simulink model "PWM_controller"  (R2014b)
settings: Solver=FixedStepDiscrete  StartTime=0.0  StopTime=150000  FixedStep=1  RelTol=1e-3
libraries: simulink x1
settings Model: FPTRunName=FPA_Reference  SimulationMode=rapid-accelerator  Creator=variable  LastModifiedBy=maclab3
settings DataIOCC: SaveOutput=off  SignalLogging=off  DSMLogging=off  SaveTime=off
settings OptimizationCC: BlockReduction=off  ConditionallyExecuteInputs=off  InlineParams=on
settings DebuggingCC: SignalRangeChecking=warning  AlgebraicLoopMsg=error  ParameterDowncastMsg=warning  ParameterOverflowMsg=warning  LoggingUnavailableSignals=none
settings HardwareCC: ProdHWDeviceType=ASIC/FPGA->ASIC/FPGA  TargetLongLongMode=on  TargetIntDivRoundTo=Zero  TargetEndianess=LittleEndian  TargetHWDeviceType=MATLAB Host  ProdEqTarget=off

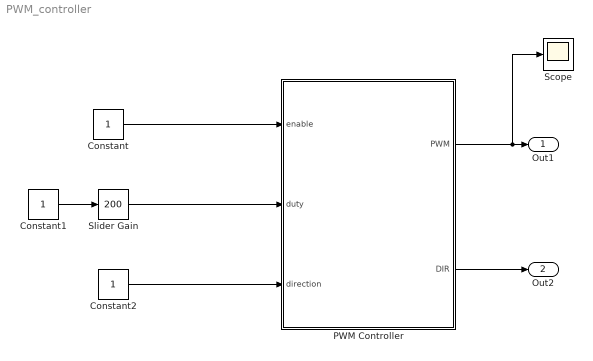
== system PWM_controller ==
  Constant : Constant  OutDataTypeStr=boolean  SampleTime=-1
  Constant1 : Constant  OutDataTypeStr=uint8  SampleTime=-1
  Constant2 : Constant  OutDataTypeStr=boolean  SampleTime=-1
  PWM Controller : Subsystem  TreatAsAtomicUnit=on
  Scope : Scope
  Slider Gain : simulink/Math Operations/Slider Gain  low=0  gain=200  high=255
  Out1 : Outport
  Out2 : Outport  Port=2
  wires:
  Constant/1 -> PWM Controller/1(enable)
  Constant1/1 -> Slider Gain/1
  Constant2/1 -> PWM Controller/3(direction)
  Slider Gain/1 -> PWM Controller/2(duty)
  PWM Controller/1(PWM) -> Scope/1, Out1/1
  PWM Controller/2(DIR) -> Out2/1

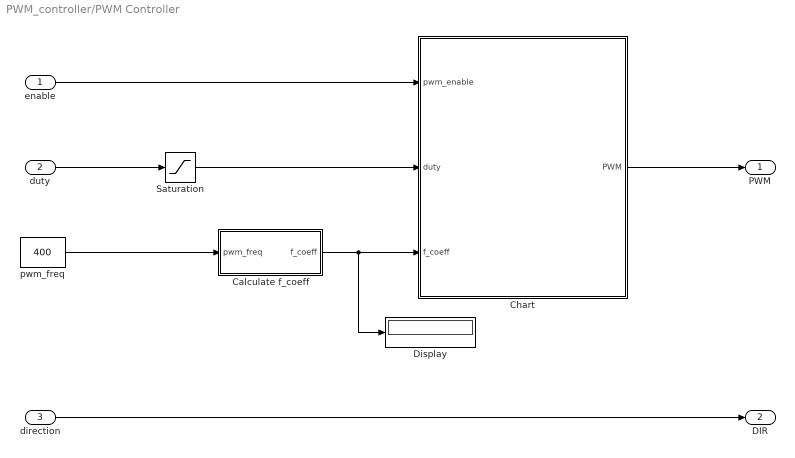
== system PWM_controller/PWM Controller ==
  enable : Inport
  duty : Inport  Port=2  OutDataTypeStr=fixdt(0,8,0)
  direction : Inport  Port=3
  Calculate f_coeff : Subsystem  TreatAsAtomicUnit=on
  Chart : Stateflow chart  TreatAsAtomicUnit=on
  Display : Display
  Saturation : Saturate  UpperLimit=255  LowerLimit=0  OutDataTypeStr=fixdt(0,8,0)
  pwm_freq : Constant  Value=400  OutDataTypeStr=uint32
  PWM : Outport
  DIR : Outport  Port=2
  wires:
  Calculate f_coeff/1(f_coeff) -> Display/1, Chart/3(f_coeff)
  Chart/1(PWM) -> PWM/1
  duty/1 -> Saturation/1
  pwm_freq/1 -> Calculate f_coeff/1(pwm_freq)
  direction/1 -> DIR/1
  Saturation/1 -> Chart/2(duty)
  enable/1 -> Chart/1(pwm_enable)

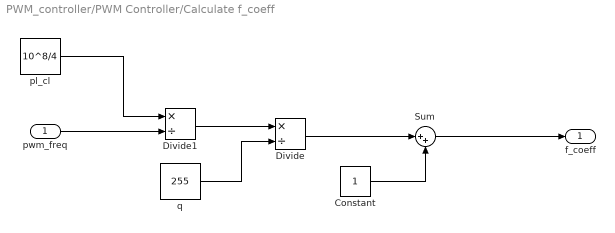
== system PWM_controller/PWM Controller/Calculate f_coeff ==
  pwm_freq : Inport
  Constant : Constant  OutDataTypeStr=uint32
  Divide : Product  Inputs=*/  SaturateOnIntegerOverflow=on  RndMeth=Zero
  Divide1 : Product  Inputs=*/  SaturateOnIntegerOverflow=on  RndMeth=Zero
  Sum : Sum  Inputs=|++  AccumDataTypeStr=uint32  RndMeth=Zero
  pl_cl : Constant  Value=10^8/4  OutDataTypeStr=uint32
  q : Constant  Value=255  OutDataTypeStr=Inherit: Inherit via back propagation
  f_coeff : Outport  OutDataTypeStr=uint32
  wires:
  q/1 -> Divide/2
  Divide1/1 -> Divide/1
  pwm_freq/1 -> Divide1/2
  pl_cl/1 -> Divide1/1
  Divide/1 -> Sum/1
  Sum/1 -> f_coeff/1
  Constant/1 -> Sum/2

== stateflow chart PWM_controller/PWM Controller/Chart ==
  settings: executeAtInitialization=1
  state S1
  note: The multiple of 40 for f_coeff raises the counts to 10,200 for one PWM wave, resulting in a frequency of 9804 Hz
      | Max PWM Frequency for the Cytron is 10 KHz
  state LOW
  state HIGH
  state S2
  (default) -> S1
  S2 -> S1
  S1 -> LOW : [pwm_enable == 1]{count = uint16(0); PWM = false;}
  LOW -> LOW [order 2] : {count = count + 1;}
  HIGH -> HIGH [order 3] : {count = count + 1;}
  LOW -> HIGH [order 1] : [count >= uint32(255-duty)*f_coeff && duty > 0]{PWM = true;}
  HIGH -> LOW [order 1] : [count >= uint32(255)*f_coeff && duty < 255]
      | {PWM = false; count = uint16(0);}
  LOW -> S2 [order 3] : [pwm_enable == 0]{PWM=false}
  HIGH -> S2 [order 2] : [pwm_enable == 0]{PWM = false;}
  data: PWM output boolean [0..1]; pwm_enable input [0..1]; count local; duty input; f_coeff input
